simulink library "PE_components"  (R2019b)
settings: Solver=VariableStepAuto  StartTime=0.0  StopTime=10.0  RelTol=1e-3
undefined symbols (not defined in the file): j, kszi0, L, Ld, Lq, pp, Rs, Theta
libraries: coordinate_transformations x18, simulink x1
settings Model: Creator=kissd  LastModifiedBy=kissd

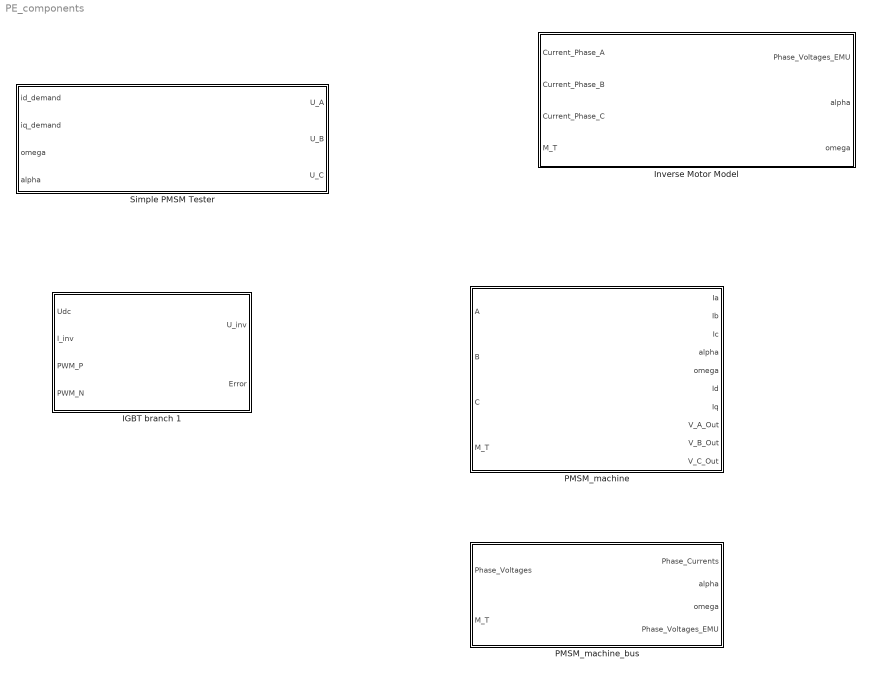
== system PE_components ==
  IGBT branch 1 : Subsystem
  Inverse Motor Model : Subsystem
  PMSM_machine : Subsystem
  PMSM_machine_bus : Subsystem  AncestorBlock=PE_components/PMSM_machine
  Simple PMSM Tester : Subsystem

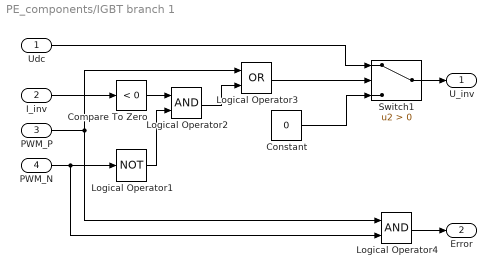
== system PE_components/IGBT branch 1 ==
  Udc : Inport
  I_inv : Inport  Port=2
  PWM_P : Inport  Port=3
  PWM_N : Inport  Port=4
  Compare To Zero : simulink/Logic and Bit Operations/Compare To Zero  relop=<  OutDataTypeStr=boolean
  Constant : Constant  Value=0
  Logical Operator1 : Logic  Operator=NOT  AllPortsSameDT=off  OutDataTypeStr=boolean
  Logical Operator2 : Logic  AllPortsSameDT=off  OutDataTypeStr=boolean
  Logical Operator3 : Logic  Operator=OR  AllPortsSameDT=off  OutDataTypeStr=boolean
  Logical Operator4 : Logic  AllPortsSameDT=off  OutDataTypeStr=boolean
  Switch1 : Switch  Criteria=u2 > Threshold
  U_inv : Outport
  Error : Outport  Port=2  OutDataTypeStr=boolean
  wires:
  Constant/1 -> Switch1/3
  Logical Operator3/1 -> Switch1/2
  PWM_N/1 -> Logical Operator4/2, Logical Operator1/1
  Logical Operator4/1 -> Error/1
  I_inv/1 -> Compare To Zero/1
  PWM_P/1 -> Logical Operator4/1, Logical Operator3/1
  Switch1/1 -> U_inv/1
  Logical Operator2/1 -> Logical Operator3/2
  Logical Operator1/1 -> Logical Operator2/2
  Udc/1 -> Switch1/1
  Compare To Zero/1 -> Logical Operator2/1

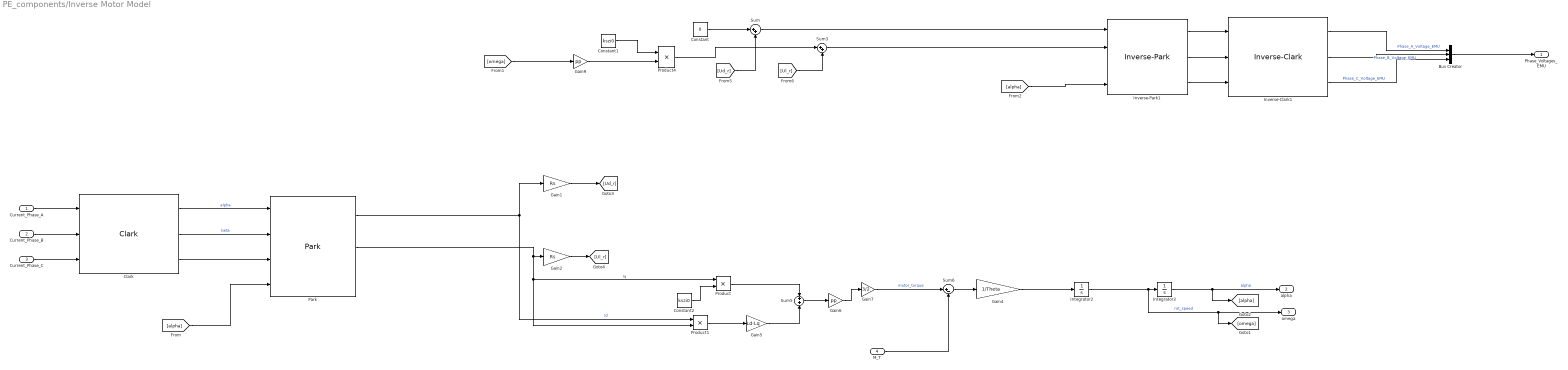
== system PE_components/Inverse Motor Model ==
  Current_Phase_A : Inport
  Current_Phase_B : Inport  Port=2
  Current_Phase_C : Inport  Port=3
  M_T : Inport  Port=4
  Bus Creator : BusCreator  Inputs=3
  Clark : coordinate_transformations/Clark  SystemSampleTime=-1  Latency=0  AutoFrameSizeCalculation=off
  Constant : Constant  Value=0
  Constant1 : Constant  Value=kszi0
  Constant2 : Constant  Value=kszi0
  Gain1 : Gain  Gain=Rs
  Gain2 : Gain  Gain=Rs
  Gain4 : Gain  Gain=1/Theta
  Gain5 : Gain  Gain=Ld-Lq
  Gain6 : Gain  Gain=pp
  Gain7 : Gain  Gain=3/2
  Gain9 : Gain  Gain=pp
  Integrator2 : Integrator
  Integrator3 : Integrator
  Inverse-Clark1 : coordinate_transformations/Inverse-Clark  SystemSampleTime=-1  Latency=0  AutoFrameSizeCalculation=off
  Inverse-Park1 : coordinate_transformations/Inverse-Park  SystemSampleTime=-1  Latency=0  AutoFrameSizeCalculation=off
  Park : coordinate_transformations/Park  SystemSampleTime=-1  Latency=0  AutoFrameSizeCalculation=off
  Product : Product
  Product1 : Product
  Product4 : Product
  Sum : Sum  Inputs=|++
  Sum3 : Sum  Inputs=|++
  Sum5 : Sum  Inputs=+|+
  Sum6 : Sum  Inputs=|+-
  Phase_Voltages_EMU : Outport
  alpha : Outport  Port=2
  omega : Outport  Port=3
  wires:
  Inverse-Clark1/2 -> Bus Creator/2  "Phase_B_Voltage_EMU"
  Current_Phase_A/1 -> Clark/1
  Clark/3 -> Park/3
  [Ud_r] -> Sum/2
  Inverse-Park1/2 -> Inverse-Clark1/2
  Gain9/1 -> Product4/2
  Current_Phase_C/1 -> Clark/3
  Integrator2/1 -> Integrator3/1, omega/1, [omega]  "rot_speed"
  Park/2 -> Product1/2, Product/1, Gain2/1  "Iq"
  Product4/1 -> Sum3/1
  Product/1 -> Sum5/1
  [alpha] -> Inverse-Park1/4
  Gain6/1 -> Gain7/1
  Inverse-Clark1/1 -> Bus Creator/1  "Phase_A_Voltage_EMU"
  Constant2/1 -> Product/2
  Sum5/1 -> Gain6/1
  Park/1 -> Gain1/1, Product1/1  "Id"
  Integrator3/1 -> alpha/1, [alpha]  "alpha"
  [alpha] -> Park/4
  Clark/2 -> Park/2  "beta"
  M_T/1 -> Sum6/2
  [omega] -> Gain9/1
  Current_Phase_B/1 -> Clark/2
  Inverse-Clark1/3 -> Bus Creator/3  "Phase_C_Voltage_EMU"
  Inverse-Park1/1 -> Inverse-Clark1/1
  Gain1/1 -> [Ud_r]
  Gain4/1 -> Integrator2/1
  Product1/1 -> Gain5/1
  [Ul_r] -> Sum3/2
  Sum3/1 -> Inverse-Park1/2
  Sum/1 -> Inverse-Park1/1
  Gain7/1 -> Sum6/1  "motor_torque"
  Inverse-Park1/3 -> Inverse-Clark1/3
  Gain2/1 -> [Ul_r]
  Bus Creator/1 -> Phase_Voltages_EMU/1
  Sum6/1 -> Gain4/1
  Gain5/1 -> Sum5/2
  Constant/1 -> Sum/1
  Clark/1 -> Park/1  "alpha"
  Constant1/1 -> Product4/1

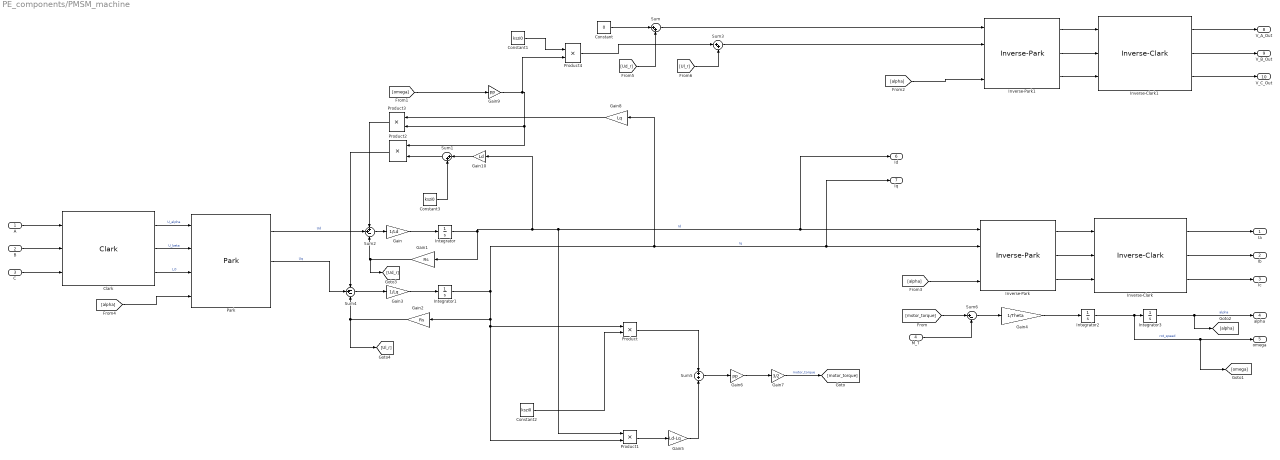
== system PE_components/PMSM_machine ==
  A : Inport
  B : Inport  Port=2
  C : Inport  Port=3
  M_T : Inport  Port=4
  Clark : coordinate_transformations/Clark  SystemSampleTime=-1  Latency=0  AutoFrameSizeCalculation=off
  Constant : Constant  Value=0
  Constant1 : Constant  Value=kszi0
  Constant2 : Constant  Value=kszi0
  Constant3 : Constant  Value=kszi0
  Gain : Gain  Gain=1/Ld
  Gain1 : Gain  Gain=Rs
  Gain10 : Gain  Gain=Ld
  Gain2 : Gain  Gain=Rs
  Gain3 : Gain  Gain=1/Lq
  Gain4 : Gain  Gain=1/Theta
  Gain5 : Gain  Gain=Ld-Lq
  Gain6 : Gain  Gain=pp
  Gain7 : Gain  Gain=3/2
  Gain8 : Gain  Gain=Lq
  Gain9 : Gain  Gain=pp
  Integrator{,1..3} (4 alike) : Integrator
  Inverse-Clark : coordinate_transformations/Inverse-Clark  SystemSampleTime=-1  Latency=0  AutoFrameSizeCalculation=off
  Inverse-Clark1 : coordinate_transformations/Inverse-Clark  SystemSampleTime=-1  Latency=0  AutoFrameSizeCalculation=off
  Inverse-Park : coordinate_transformations/Inverse-Park  SystemSampleTime=-1  Latency=0  AutoFrameSizeCalculation=off
  Inverse-Park1 : coordinate_transformations/Inverse-Park  SystemSampleTime=-1  Latency=0  AutoFrameSizeCalculation=off
  Park : coordinate_transformations/Park  SystemSampleTime=-1  Latency=0  AutoFrameSizeCalculation=off
  Product{,1..4} (5 alike) : Product
  Sum : Sum  Inputs=|++
  Sum1 : Sum  Inputs=|++
  Sum2 : Sum  Inputs=++-
  Sum3 : Sum  Inputs=|++
  Sum4 : Sum  Inputs=-+-
  Sum5 : Sum  Inputs=+|+
  Sum6 : Sum  Inputs=|+-
  Ia : Outport
  Ib : Outport  Port=2
  Ic : Outport  Port=3
  alpha : Outport  Port=4
  omega : Outport  Port=5
  Id : Outport  Port=6
  "Iq " : Outport  Port=7
  V_A_Out : Outport  Port=8
  V_B_Out : Outport  Port=9
  V_C_Out : Outport  Port=10
  wires:
  A/1 -> Clark/1
  B/1 -> Clark/2
  C/1 -> Clark/3
  Clark/1 -> Park/1  "U_alpha"
  Clark/2 -> Park/2  "U_beta"
  Clark/3 -> Park/3  "I_0"
  Inverse-Clark/1 -> Ia/1
  Inverse-Clark/2 -> Ib/1
  Inverse-Clark/3 -> Ic/1
  Inverse-Park/1 -> Inverse-Clark/1
  Inverse-Park/2 -> Inverse-Clark/2
  Inverse-Park/3 -> Inverse-Clark/3
  Park/1 -> Sum2/2  "Ud"
  Gain/1 -> Integrator/1
  Integrator/1 -> Gain1/1, Gain10/1, Product1/1, Id/1, Inverse-Park/1  "Id"
  Gain3/1 -> Integrator1/1
  Gain2/1 -> Sum4/3, [Ul_r]
  Park/2 -> Sum4/2  "Uq"
  Sum4/1 -> Gain3/1
  Integrator1/1 -> Gain8/1, "Iq "/1, Inverse-Park/2, Product/1, Product1/2, Gain2/1  "Iq"
  Constant2/1 -> Product/2
  Product1/1 -> Gain5/1
  Product/1 -> Sum5/1
  Gain5/1 -> Sum5/2
  Sum5/1 -> Gain6/1
  Gain6/1 -> Gain7/1
  Gain7/1 -> [motor_torque]  "motor_torque"
  [motor_torque] -> Sum6/1
  M_T/1 -> Sum6/2
  Sum2/1 -> Gain/1
  Gain1/1 -> [Ud_r], Sum2/3
  [omega] -> Gain9/1
  Product3/1 -> Sum2/1
  Gain8/1 -> Product3/1
  Gain9/1 -> Product4/2, Product2/1, Product3/2
  Sum1/1 -> Product2/2
  Gain10/1 -> Sum1/1
  Constant3/1 -> Sum1/2
  Product2/1 -> Sum4/1
  Sum6/1 -> Gain4/1
  Gain4/1 -> Integrator2/1
  Integrator2/1 -> [omega], omega/1, Integrator3/1  "rot_speed"
  Integrator3/1 -> [alpha], alpha/1  "alpha"
  [alpha] -> Park/4
  [alpha] -> Inverse-Park/4
  Inverse-Park1/2 -> Inverse-Clark1/2
  Inverse-Clark1/3 -> V_C_Out/1
  Inverse-Park1/1 -> Inverse-Clark1/1
  Inverse-Park1/3 -> Inverse-Clark1/3
  Inverse-Clark1/1 -> V_A_Out/1
  [alpha] -> Inverse-Park1/4
  Inverse-Clark1/2 -> V_B_Out/1
  Sum/1 -> Inverse-Park1/1
  Sum3/1 -> Inverse-Park1/2
  [Ud_r] -> Sum/2
  [Ul_r] -> Sum3/2
  Constant/1 -> Sum/1
  Constant1/1 -> Product4/1
  Product4/1 -> Sum3/1

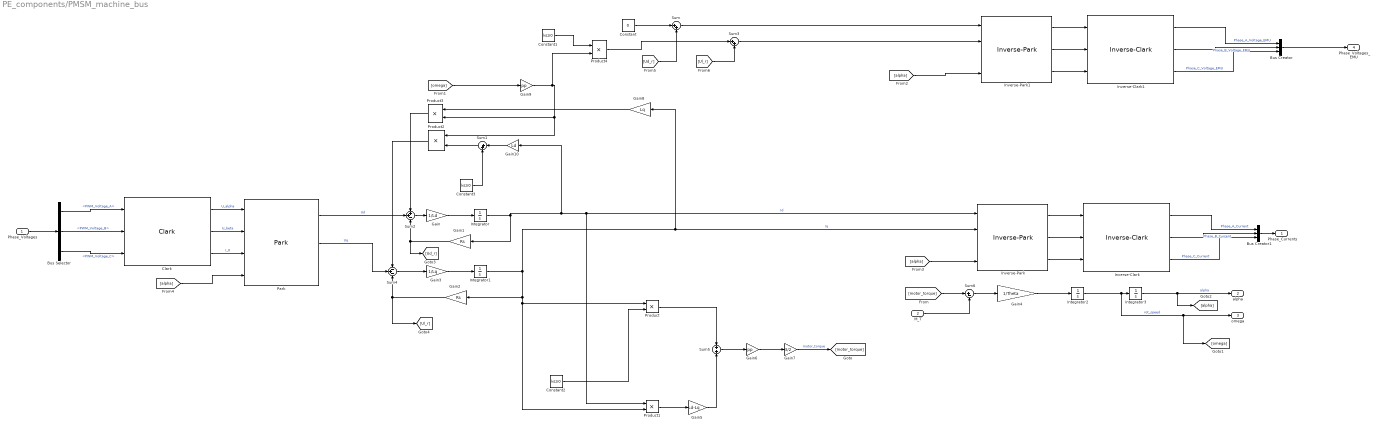
== system PE_components/PMSM_machine_bus ==
  Phase_Voltages : Inport
  M_T : Inport  Port=2
  Bus Creator : BusCreator  Inputs=3
  Bus Creator1 : BusCreator  Inputs=3
  Bus Selector : BusSelector  OutputSignals=PWM_Voltage_A,PWM_Voltage_B,PWM_Voltage_C
  Clark : coordinate_transformations/Clark  SystemSampleTime=-1  Latency=0  AutoFrameSizeCalculation=off
  Constant : Constant  Value=0
  Constant1 : Constant  Value=kszi0
  Constant2 : Constant  Value=kszi0
  Constant3 : Constant  Value=kszi0
  Gain : Gain  Gain=1/Ld
  Gain1 : Gain  Gain=Rs
  Gain10 : Gain  Gain=Ld
  Gain2 : Gain  Gain=Rs
  Gain3 : Gain  Gain=1/Lq
  Gain4 : Gain  Gain=1/Theta
  Gain5 : Gain  Gain=Ld-Lq
  Gain6 : Gain  Gain=pp
  Gain7 : Gain  Gain=3/2
  Gain8 : Gain  Gain=Lq
  Gain9 : Gain  Gain=pp
  Integrator{,1..3} (4 alike) : Integrator
  Inverse-Clark : coordinate_transformations/Inverse-Clark  SystemSampleTime=-1  Latency=0  AutoFrameSizeCalculation=off
  Inverse-Clark1 : coordinate_transformations/Inverse-Clark  SystemSampleTime=-1  Latency=0  AutoFrameSizeCalculation=off
  Inverse-Park : coordinate_transformations/Inverse-Park  SystemSampleTime=-1  Latency=0  AutoFrameSizeCalculation=off
  Inverse-Park1 : coordinate_transformations/Inverse-Park  SystemSampleTime=-1  Latency=0  AutoFrameSizeCalculation=off
  Park : coordinate_transformations/Park  SystemSampleTime=-1  Latency=0  AutoFrameSizeCalculation=off
  Product{,1..4} (5 alike) : Product
  Sum : Sum  Inputs=|++
  Sum1 : Sum  Inputs=|++
  Sum2 : Sum  Inputs=++-
  Sum3 : Sum  Inputs=|++
  Sum4 : Sum  Inputs=-+-
  Sum5 : Sum  Inputs=+|+
  Sum6 : Sum  Inputs=|+-
  Phase_Currents : Outport
  alpha : Outport  Port=2
  omega : Outport  Port=3
  Phase_Voltages_EMU : Outport  Port=4
  wires:
  Product4/1 -> Sum3/1
  Constant1/1 -> Product4/1
  Constant/1 -> Sum/1
  [Ul_r] -> Sum3/2
  [Ud_r] -> Sum/2
  Sum3/1 -> Inverse-Park1/2
  Sum/1 -> Inverse-Park1/1
  Inverse-Clark1/2 -> Bus Creator/2  "Phase_B_Voltage_EMU"
  [alpha] -> Inverse-Park1/4
  Inverse-Clark1/1 -> Bus Creator/1  "Phase_A_Voltage_EMU"
  Inverse-Park1/3 -> Inverse-Clark1/3
  Inverse-Park1/1 -> Inverse-Clark1/1
  Inverse-Clark1/3 -> Bus Creator/3  "Phase_C_Voltage_EMU"
  Inverse-Park1/2 -> Inverse-Clark1/2
  [alpha] -> Inverse-Park/4
  [alpha] -> Park/4
  Integrator3/1 -> alpha/1, [alpha]  "alpha"
  Integrator2/1 -> Integrator3/1, omega/1, [omega]  "rot_speed"
  Gain4/1 -> Integrator2/1
  Sum6/1 -> Gain4/1
  Product2/1 -> Sum4/1
  Constant3/1 -> Sum1/2
  Gain10/1 -> Sum1/1
  Sum1/1 -> Product2/2
  Gain9/1 -> Product3/2, Product2/1, Product4/2
  Gain8/1 -> Product3/1
  Product3/1 -> Sum2/1
  [omega] -> Gain9/1
  Gain1/1 -> Sum2/3, [Ud_r]
  Sum2/1 -> Gain/1
  M_T/1 -> Sum6/2
  [motor_torque] -> Sum6/1
  Gain7/1 -> [motor_torque]  "motor_torque"
  Gain6/1 -> Gain7/1
  Sum5/1 -> Gain6/1
  Gain5/1 -> Sum5/2
  Product/1 -> Sum5/1
  Product1/1 -> Gain5/1
  Constant2/1 -> Product/2
  Integrator1/1 -> Gain2/1, Product1/2, Product/1, Inverse-Park/2, Gain8/1  "Iq"
  Sum4/1 -> Gain3/1
  Park/2 -> Sum4/2  "Uq"
  Gain2/1 -> [Ul_r], Sum4/3
  Gain3/1 -> Integrator1/1
  Integrator/1 -> Inverse-Park/1, Product1/1, Gain10/1, Gain1/1  "Id"
  Gain/1 -> Integrator/1
  Park/1 -> Sum2/2  "Ud"
  Inverse-Park/3 -> Inverse-Clark/3
  Inverse-Park/2 -> Inverse-Clark/2
  Inverse-Park/1 -> Inverse-Clark/1
  Inverse-Clark/3 -> Bus Creator1/3  "Phase_C_Current"
  Inverse-Clark/2 -> Bus Creator1/2  "Phase_B_Current"
  Inverse-Clark/1 -> Bus Creator1/1  "Phase_A_Current"
  Clark/3 -> Park/3  "I_0"
  Clark/2 -> Park/2  "U_beta"
  Clark/1 -> Park/1  "U_alpha"
  Phase_Voltages/1 -> Bus Selector/1
  Bus Selector/1 -> Clark/1  "<PWM_Voltage_A>"
  Bus Selector/2 -> Clark/2  "<PWM_Voltage_B>"
  Bus Selector/3 -> Clark/3  "<PWM_Voltage_C>"
  Bus Creator/1 -> Phase_Voltages_EMU/1
  Bus Creator1/1 -> Phase_Currents/1

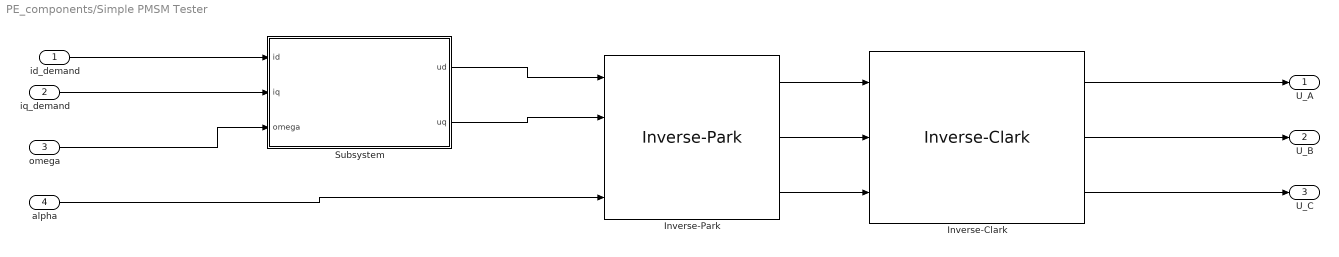
== system PE_components/Simple PMSM Tester ==
  id_demand : Inport
  iq_demand : Inport  Port=2
  omega : Inport  Port=3
  alpha : Inport  Port=4
  Inverse-Clark : coordinate_transformations/Inverse-Clark  SystemSampleTime=-1  Latency=0  AutoFrameSizeCalculation=off
  Inverse-Park : coordinate_transformations/Inverse-Park  SystemSampleTime=-1  Latency=0  AutoFrameSizeCalculation=off
  Subsystem : Subsystem
  U_A : Outport
  U_B : Outport  Port=2
  U_C : Outport  Port=3
  wires:
  Inverse-Park/2 -> Inverse-Clark/2
  Subsystem/2(uq) -> Inverse-Park/2
  Inverse-Park/1 -> Inverse-Clark/1
  Inverse-Clark/2 -> U_B/1
  Subsystem/1(ud) -> Inverse-Park/1
  omega/1 -> Subsystem/3(omega)
  Inverse-Park/3 -> Inverse-Clark/3
  iq_demand/1 -> Subsystem/2("iq ")
  Inverse-Clark/3 -> U_C/1
  Inverse-Clark/1 -> U_A/1
  alpha/1 -> Inverse-Park/4
  id_demand/1 -> Subsystem/1(id)

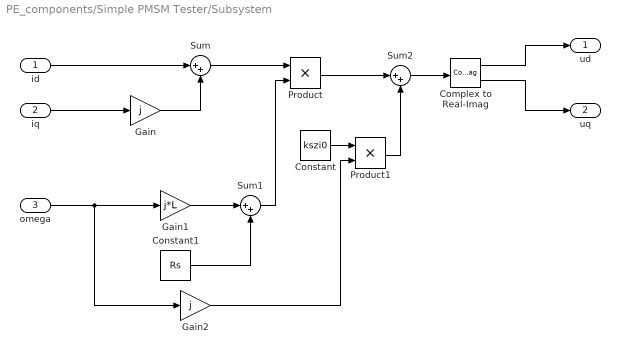
== system PE_components/Simple PMSM Tester/Subsystem ==
  id : Inport
  "iq " : Inport  Port=2
  omega : Inport  Port=3
  Complex to Real-Imag : ComplexToRealImag
  Constant : Constant  Value=kszi0
  Constant1 : Constant  Value=Rs
  Gain : Gain  Gain=j
  Gain1 : Gain  Gain=j*L
  Gain2 : Gain  Gain=j
  Product : Product
  Product1 : Product
  Sum : Sum  Inputs=|++
  Sum1 : Sum  Inputs=|++
  Sum2 : Sum  Inputs=|++
  ud : Outport
  uq : Outport  Port=2
  wires:
  "iq "/1 -> Gain/1
  id/1 -> Sum/1
  Gain/1 -> Sum/2
  omega/1 -> Gain2/1, Gain1/1
  Gain1/1 -> Sum1/1
  Constant1/1 -> Sum1/2
  Sum1/1 -> Product/2
  Sum/1 -> Product/1
  Product/1 -> Sum2/1
  Constant/1 -> Product1/1
  Gain2/1 -> Product1/2
  Product1/1 -> Sum2/2
  Sum2/1 -> Complex to Real-Imag/1
  Complex to Real-Imag/1 -> ud/1
  Complex to Real-Imag/2 -> uq/1
